simulink model "rlFlyingRobotEnv"  (R2022b)
settings: Solver=VariableStepAuto  StartTime=0.0  StopTime=10.0  RelTol=1e-3
values from neighbouring files (symbols this model uses):
  theta0 = 0    [TrainDDPGAgentToControlFlyingRobotExample.m]    (also in TrainDDPGAgentToControlFlyingRobotExamplePPO.m)
  Ts = 0.4    [TrainDDPGAgentToControlFlyingRobotExample.m]    (also in TrainDDPGAgentToControlFlyingRobotExamplePPO.m)
  x0 = -15    [TrainDDPGAgentToControlFlyingRobotExample.m]    (also in TrainDDPGAgentToControlFlyingRobotExamplePPO.m; flyingRobotResetFcn.m = cos(t1)*R)
  xmax = 60    [TrainDDPGAgentToControlFlyingRobotExamplePPO.m]
  y0 = 0    [TrainDDPGAgentToControlFlyingRobotExample.m]    (also in TrainDDPGAgentToControlFlyingRobotExamplePPO.m; flyingRobotResetFcn.m = sin(t1)*R)
  ymax = 60    [TrainDDPGAgentToControlFlyingRobotExamplePPO.m]
libraries: simulink x3
settings Model: Creator=The MathWorks, Inc.  LastModifiedBy=spenc
settings SolverCC: AlgebraicLoopSolver=TrustRegion
settings DataIOCC: ReturnWorkspaceOutputs=off
settings DebuggingCC: UnconnectedInputMsg=warning  UnconnectedOutputMsg=warning  UnconnectedLineMsg=warning  SFMachineParentedDataDiag=warning  ArithmeticOperatorsInVariantConditions=warning
settings ModelReferenceCC: EnableRefExpFcnMdlSchedulingChecks=on  ModelReferenceMinAlgLoopOccurrences=on

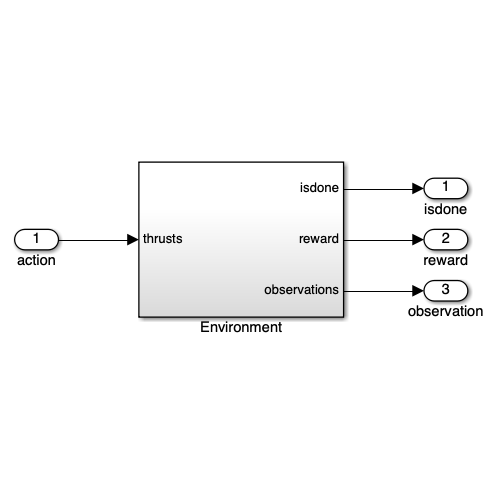
[thumbnail: Simulink's stored preview of the top-level diagram]
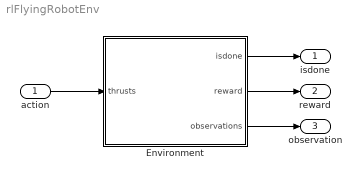
== system rlFlyingRobotEnv ==
  action : Inport
  Environment : Subsystem
  isdone : Outport  VectorParamsAs1DForOutWhenUnconnected=off
  reward : Outport  Port=2  VectorParamsAs1DForOutWhenUnconnected=off
  observation : Outport  Port=3  VectorParamsAs1DForOutWhenUnconnected=off
  wires:
  Environment/3(observations) -> observation/1
  Environment/2(reward) -> reward/1
  Environment/1(isdone) -> isdone/1
  action/1 -> Environment/1(thrusts)

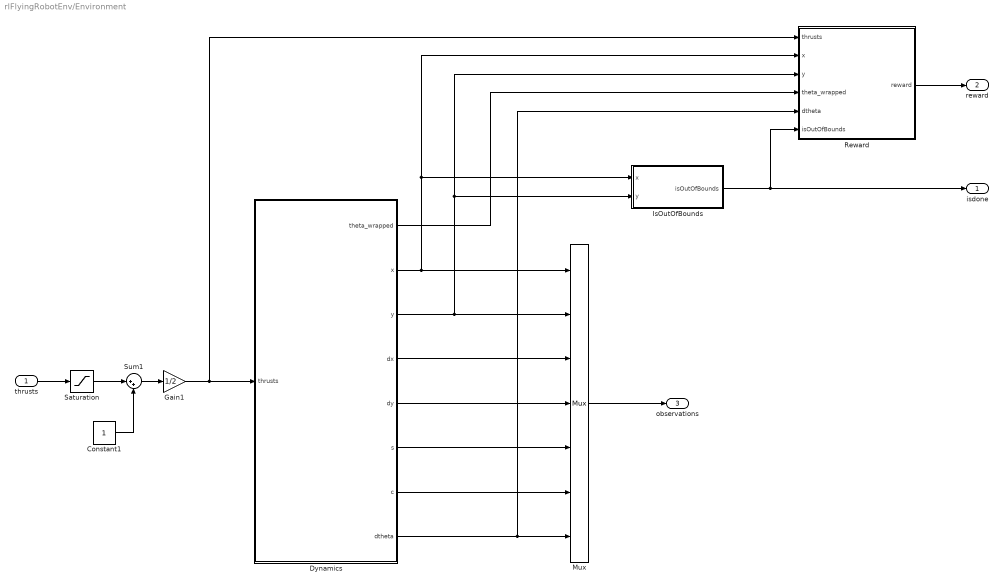
== system rlFlyingRobotEnv/Environment ==
  thrusts : Inport
  Constant1 : Constant
  Dynamics : Subsystem
  Gain1 : Gain  Gain=1/2
  IsOutOfBounds : Subsystem
  Mux : Mux  Inputs=7
  Reward : Subsystem
  Saturation : Saturate  UpperLimit=1  LowerLimit=-1
  Sum1 : Sum  Inputs=|++
  isdone : Outport  VectorParamsAs1DForOutWhenUnconnected=off
  reward : Outport  Port=2  VectorParamsAs1DForOutWhenUnconnected=off
  observations : Outport  Port=3  VectorParamsAs1DForOutWhenUnconnected=off
  wires:
  Reward/1(reward) -> reward/1
  IsOutOfBounds/1(isOutOfBounds) -> isdone/1, Reward/6(isOutOfBounds)
  Dynamics/1(theta_wrapped) -> Reward/4(theta_wrapped)
  Dynamics/3(y) -> Mux/2, IsOutOfBounds/2(y), Reward/3(y)
  Dynamics/2(x) -> Mux/1, IsOutOfBounds/1(x), Reward/2(x)
  Mux/1 -> observations/1
  Gain1/1 -> Reward/1(thrusts), Dynamics/1(thrusts)
  thrusts/1 -> Saturation/1
  Dynamics/4(dx) -> Mux/3
  Dynamics/5(dy) -> Mux/4
  Dynamics/6(s) -> Mux/5
  Dynamics/7(c) -> Mux/6
  Dynamics/8(dtheta) -> Reward/5(dtheta), Mux/7
  Saturation/1 -> Sum1/1
  Sum1/1 -> Gain1/1
  Constant1/1 -> Sum1/2

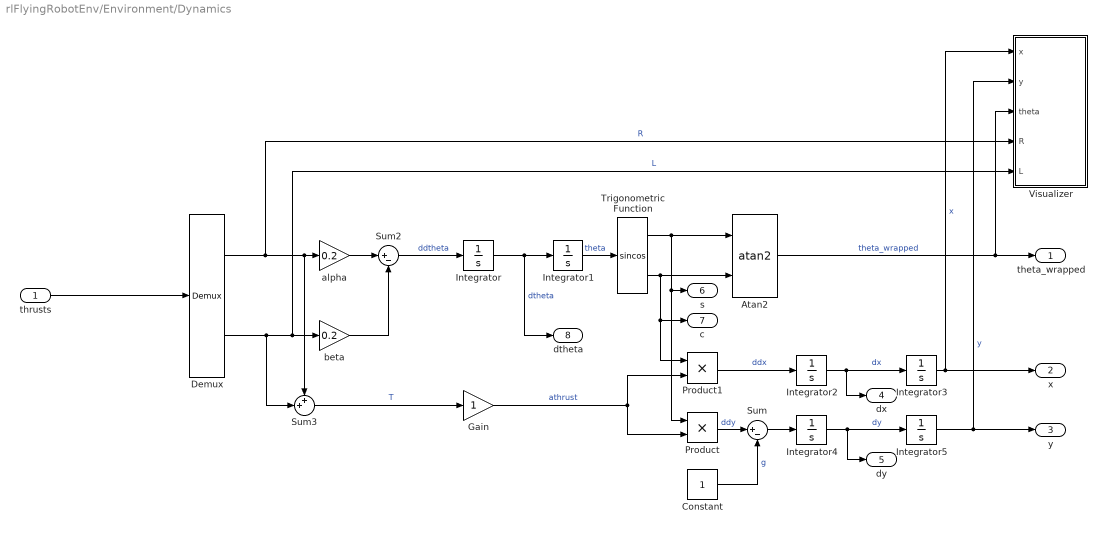
== system rlFlyingRobotEnv/Environment/Dynamics ==
  thrusts : Inport
  Atan2 : Trigonometry  Operator=atan2
  Constant : Constant
  Demux : Demux  Outputs=2
  Gain : Gain
  Integrator : Integrator
  Integrator1 : Integrator  InitialCondition=theta0
  Integrator2 : Integrator
  Integrator3 : Integrator  InitialCondition=x0
  Integrator4 : Integrator
  Integrator5 : Integrator  InitialCondition=y0
  Product : Product
  Product1 : Product
  Sum : Sum  Inputs=|+-
  Sum2 : Sum  Inputs=|+-
  Sum3 : Sum  Inputs=++|
  Trigonometric Function : Trigonometry  Operator=sincos
  Visualizer : Subsystem
  alpha : Gain  Gain=0.2
  beta : Gain  Gain=0.2
  theta_wrapped : Outport  VectorParamsAs1DForOutWhenUnconnected=off
  x : Outport  Port=2  VectorParamsAs1DForOutWhenUnconnected=off
  y : Outport  Port=3  VectorParamsAs1DForOutWhenUnconnected=off
  dx : Outport  Port=4  VectorParamsAs1DForOutWhenUnconnected=off
  dy : Outport  Port=5  VectorParamsAs1DForOutWhenUnconnected=off
  s : Outport  Port=6  VectorParamsAs1DForOutWhenUnconnected=off
  c : Outport  Port=7  VectorParamsAs1DForOutWhenUnconnected=off
  dtheta : Outport  Port=8  VectorParamsAs1DForOutWhenUnconnected=off
  wires:
  Integrator1/1 -> Trigonometric Function/1  "theta"
  Product1/1 -> Integrator2/1  "ddx"
  Integrator2/1 -> dx/1, Integrator3/1  "dx"
  Demux/2 -> Sum3/2, Visualizer/5(L), beta/1  "L"
  Demux/1 -> Visualizer/4(R), Sum3/1, alpha/1  "R"
  Sum3/1 -> Gain/1  "T"
  Integrator4/1 -> Integrator5/1, dy/1  "dy"
  Trigonometric Function/1 -> s/1, Product/1, Atan2/1
  Trigonometric Function/2 -> Product1/1, c/1, Atan2/2
  Sum2/1 -> Integrator/1  "ddtheta"
  Integrator3/1 -> Visualizer/1(x), x/1  "x"
  Integrator/1 -> dtheta/1, Integrator1/1  "dtheta"
  Product/1 -> Sum/1  "ddy"
  Integrator5/1 -> Visualizer/2(y), y/1  "y"
  alpha/1 -> Sum2/1
  beta/1 -> Sum2/2
  Atan2/1 -> Visualizer/3(theta), theta_wrapped/1  "theta_wrapped"
  Sum/1 -> Integrator4/1
  Constant/1 -> Sum/2  "g"
  Gain/1 -> Product1/2, Product/2  "athrust"
  thrusts/1 -> Demux/1

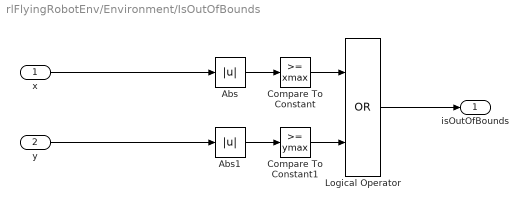
== system rlFlyingRobotEnv/Environment/IsOutOfBounds ==
  x : Inport
  y : Inport  Port=2
  Abs : Abs  SaturateOnIntegerOverflow=off
  Abs1 : Abs  SaturateOnIntegerOverflow=off
  Compare To Constant : simulink/Logic and Bit Operations/Compare To Constant  relop=>=  const=xmax  OutDataTypeStr=boolean
  Compare To Constant1 : simulink/Logic and Bit Operations/Compare To Constant  relop=>=  const=ymax  OutDataTypeStr=boolean
  Logical Operator : Logic  Operator=OR  AllPortsSameDT=off  OutDataTypeStr=boolean
  isOutOfBounds : Outport  VectorParamsAs1DForOutWhenUnconnected=off
  wires:
  Compare To Constant1/1 -> Logical Operator/2
  Compare To Constant/1 -> Logical Operator/1
  y/1 -> Abs1/1
  Abs/1 -> Compare To Constant/1
  x/1 -> Abs/1
  Abs1/1 -> Compare To Constant1/1
  Logical Operator/1 -> isOutOfBounds/1

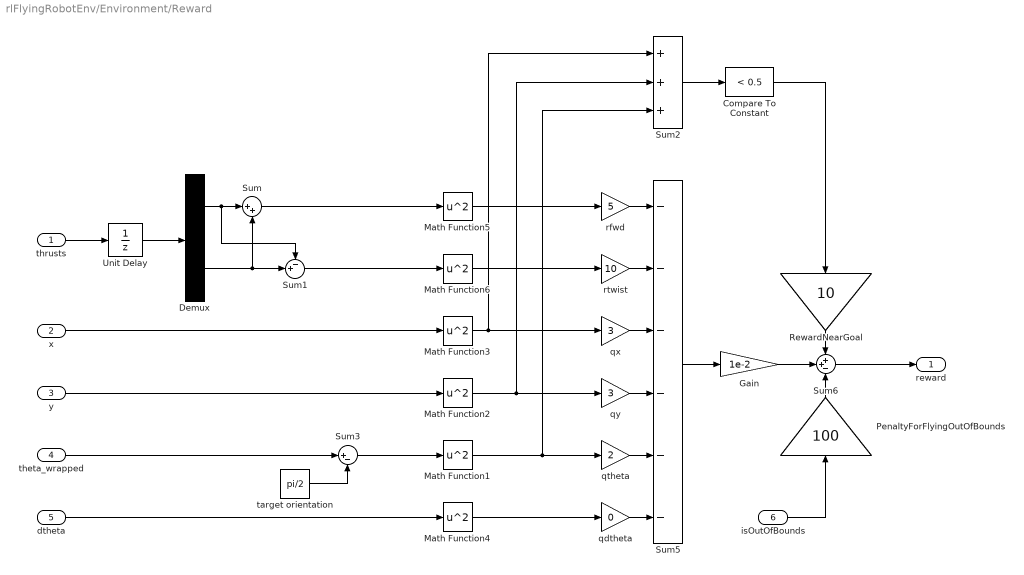
== system rlFlyingRobotEnv/Environment/Reward ==
  thrusts : Inport
  x : Inport  Port=2
  y : Inport  Port=3
  theta_wrapped : Inport  Port=4
  dtheta : Inport  Port=5
  isOutOfBounds : Inport  Port=6
  Compare To Constant : simulink/Logic and Bit Operations/Compare To Constant  relop=<  const=0.5  OutDataTypeStr=boolean
  Demux : Demux  Outputs=2
  Gain : Gain  Gain=1e-2
  Math Function{1..6} (6 alike) : Math  Operator=square  SignedPower=on
  PenaltyForFlyingOutOfBounds : Gain  Gain=100
  RewardNearGoal : Gain  Gain=10
  Sum : Sum  Inputs=|++
  Sum1 : Sum  Inputs=-+|
  Sum2 : Sum  Inputs=+++
  Sum3 : Sum  Inputs=|+-
  Sum5 : Sum  Inputs=------
  Sum6 : Sum  Inputs=++-
  Unit Delay : UnitDelay  SampleTime=Ts  HasFrameUpgradeWarning=on
  qdtheta : Gain  Gain=0
  qtheta : Gain  Gain=2
  qx : Gain  Gain=3
  qy : Gain  Gain=3
  rfwd : Gain  Gain=5
  rtwist : Gain  Gain=10
  target orientation : Constant  Value=pi/2
  reward : Outport  VectorParamsAs1DForOutWhenUnconnected=off
  wires:
  qy/1 -> Sum5/4
  qtheta/1 -> Sum5/5
  Math Function2/1 -> Sum2/2, qy/1
  Sum5/1 -> Gain/1
  theta_wrapped/1 -> Sum3/1
  Math Function1/1 -> Sum2/3, qtheta/1
  Math Function3/1 -> Sum2/1, qx/1
  rfwd/1 -> Sum5/1
  qx/1 -> Sum5/3
  thrusts/1 -> Unit Delay/1
  x/1 -> Math Function3/1
  y/1 -> Math Function2/1
  Sum6/1 -> reward/1
  isOutOfBounds/1 -> PenaltyForFlyingOutOfBounds/1
  Unit Delay/1 -> Demux/1
  Demux/1 -> Sum/1, Sum1/1
  Demux/2 -> Sum1/2, Sum/2
  Sum/1 -> Math Function5/1
  Sum1/1 -> Math Function6/1
  Math Function5/1 -> rfwd/1
  Math Function6/1 -> rtwist/1
  rtwist/1 -> Sum5/2
  qdtheta/1 -> Sum5/6
  Math Function4/1 -> qdtheta/1
  dtheta/1 -> Math Function4/1
  PenaltyForFlyingOutOfBounds/1 -> Sum6/3
  Gain/1 -> Sum6/2
  RewardNearGoal/1 -> Sum6/1
  Compare To Constant/1 -> RewardNearGoal/1
  Sum2/1 -> Compare To Constant/1
  Sum3/1 -> Math Function1/1
  target orientation/1 -> Sum3/2

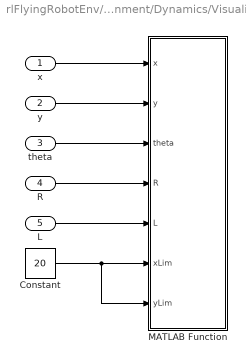
== system rlFlyingRobotEnv/Environment/Dynamics/Visualizer ==
  x : Inport
  y : Inport  Port=2
  theta : Inport  Port=3
  R : Inport  Port=4
  L : Inport  Port=5
  Constant : Constant  Value=20
  MATLAB Function : MATLAB Function  TreatAsAtomicUnit=on
  wires:
  R/1 -> MATLAB Function/4(R)
  y/1 -> MATLAB Function/2(y)
  x/1 -> MATLAB Function/1(x)
  theta/1 -> MATLAB Function/3(theta)
  Constant/1 -> MATLAB Function/7(yLim), MATLAB Function/6(xLim)
  L/1 -> MATLAB Function/5(L)

== matlab function rlFlyingRobotEnv/Environment/Dynamics/Visualizer/MATLAB Function ==
  settings: updateMethod=DISCRETE
  data: x input; y input; theta input; R input; L input; xLim input; yLim input
function fcn(x,y,theta,R,L,xLim,yLim)
%#codegen
coder.extrinsic('rl.env.viz.plotFlyingRobot');
rl.env.viz.plotFlyingRobot(x,y,theta,L,R,xLim,yLim);
